simulink model "GAModelTest"  (R2020a)
settings: Solver=FixedStepDiscrete  StartTime=0.0  StopTime=10.0  RelTol=1e-3  EnableMultiTasking=on
model workspace (MAT data in the model file):
  L1 = 0
  L2 = 0
  L3 = 0
  h1 = 0
  l1 = 0
  l2 = 0
  l3 = 0
  l4 = 0
  m1 = 0
  m2 = 0
  m3 = 0
  m4 = 0
values from neighbouring files (symbols this model uses):
  n = 2    [PolynomialFit.m]    (also in extractdata.m = 10)
undefined symbols (not defined in the file or in its folder): lb, ub
settings Model: DataDictionary=ExoskeletonParameters.sldd  Creator=khoi  LastModifiedBy=khoi
settings SolverCC: AutoInsertRateTranBlk=on
settings DataIOCC: SaveOutput=off  SaveTime=off
settings OptimizationCC: DefaultParameterBehavior=Inlined  InlineInvariantSignals=on  EnhancedBackFolding=on  PassReuseOutputArgsAs=Individual arguments  StateBitsets=on  DataBitsets=on  ZeroExternalMemoryAtStartup=off  ZeroInternalMemoryAtStartup=off  NoFixptDivByZeroProtection=on  LifeSpan=1  OptimizeBlockOrder=speed  DifferentSizesBufferReuse=on  EfficientTunableParamExpr=on
settings DebuggingCC: ParameterTunabilityLossMsg=error
settings HardwareCC: ProdBitPerPointer=32  ProdBitPerSizeT=32  ProdBitPerPtrDiffT=32  ProdLargestAtomicFloat=None  ProdIntDivRoundTo=Floor  ProdWordSize=32  ProdHWDeviceType=Generic->Custom
settings SFSimCC: MATLABDynamicMemAlloc=off
settings RTWCC: SystemTargetFile=ert.tlc  TLCOptions=-p0  GenCodeOnly=on  TemplateMakefile=ert_default_tmf  GenerateReport=on  RTWVerbose=off  IncludeHyperlinkInReport=on  LaunchReport=on
settings CodeAppCC: ForceParamTrailComments=on  IgnoreCustomStorageClasses=off  OperatorAnnotations=on  SimulinkDataObjDesc=on  SFDataObjDesc=on  CustomSymbolStrGlobalVar=rt$N$M  CustomSymbolStrType=$N$M  CustomSymbolStrFcn=$N$M$F  CustomSymbolStrMacro=$N$M  InsertBlockDesc=on
settings ERTTargetCC: TargetLangStandard=C99 (ISO)  CodeReplacementLibrary=ISO_C  GenerateSampleERTMain=on  IncludeMdlTerminateFcn=off  SuppressErrorStatus=on  SupportAbsoluteTime=off  PurelyIntegerCode=on  SupportNonFinite=off  SupportComplex=off  InlinedParameterPlacement=NonHierarchical  RootIOFormat=Structure reference  ERTCustomFileTemplate=example_file_process.tlc

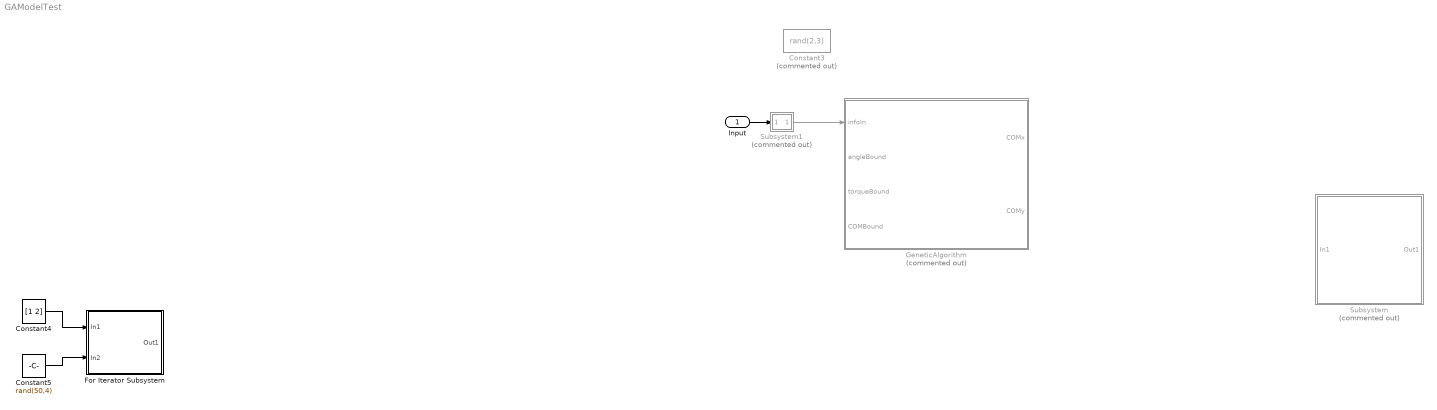
== system GAModelTest ==
  Input : Inport  OutDataTypeStr=Bus: LegSignal
  Constant3 : Constant  Commented=on  Value=rand(2,3)
  Constant4 : Constant  Value=[1 2]
  Constant5 : Constant  Value=rand(50,4)
  For Iterator Subsystem : Subsystem  InitFcn=|  TreatAsAtomicUnit=on  mask{ndec=3, anglb=[1 2 1 1], angub=[5 5 4 3], torlb=[1 1 1 1], torub=[2 2 2 2]}
      | numTotal = (ub-lb)/10^(-ndec) + 1;
      | n = floor(log2(numTotal)) + 1;
      | len = sum(n);
      mask prompts: ndec "Number of decimal place"; anglb "Lower boundary angle"; angub "Upper boundary angle"; torlb "Lower boundary torque"; torub "Upper boundary torque"
  GeneticAlgorithm : Stateflow chart  Commented=on  TreatAsAtomicUnit=on  mask{popSize=50, maxGens=200, probMutation=0.01, crossoverTypeMask=Uniform, probCrossover=0.01, ndec=3, useClamping=on, flagFreq=0, unflagFreq=0, flagPeriod=0, useMaskRepositories=on, maskReposFactor=0, useSUS=on}
      mask prompts: popSize "Population size"; maxGens "Maximum generations"; probMutation "Mutation probability (per bit)"; crossoverTypeMask "Crossover type"; probCrossover "Crossover probability"; ndec "Precision (number of decimal places)"; useClamping "Use clamping"; flagFreq "Flag frequency"; unflagFreq "Unflag frequency"; flagPeriod "Flag period"; useMaskRepositories "Use mask repositories"; maskReposFactor "Factor"; useSUS "Use Stochastic Universal Sampling"
  Subsystem : Subsystem  Commented=on  mask{gainpopup=User-defined, editvalue=2, editvalue_copy=2}
      mask prompts: gainpopup "Gain"; editvalue "Value"; editvalue_copy "Value"
      mask TypeOptions gainpopup: 2 | 5 | User-defined
      mask Callback gainpopup:
      | % Get the mask parameter values. This is a cell
      | %   array of character vectors.
      | maskStr = get_param(gcb,'gainpopup');
      | 
      | % The pop-up menu is the first mask parameter.
      | %   Check the value selected in the pop-up
      | if strcmp(maskStr(1),'U'),
      | 
      |     % Set the visibility of both parameters on when
      |     %   User-defined is selected in the pop-up.
      | 
      |     set_param(gcb,'MaskVisibilities',{'on';'on'}),
      | 
      | else
      | 
      |     % Turn off the visibility of the Value field
      |     %   when User-defined is not selected.
      | 
      |     set_param(gcb,'MaskVisibilities',{'on';'off'}),
      | 
      |     % Set the character vector in the Values field equal to the
      |     % character vector selected in the Gain pop-up menu.
      | 
      |     %maskStr{2}=maskStr{1};
      |     set_param(gcb,'editvalue',maskStr);
      | %     set_param(gcb,'editvalue1',maskStr);
      | end
  Subsystem1 : Subsystem  Commented=on
  wires:
  Input/1 -> Subsystem1/1(In1)
  Subsystem1/1(Out1) -> GeneticAlgorithm/1(infoIn)
  Constant4/1 -> For Iterator Subsystem/1(In1)
  Constant5/1 -> For Iterator Subsystem/2(In2)

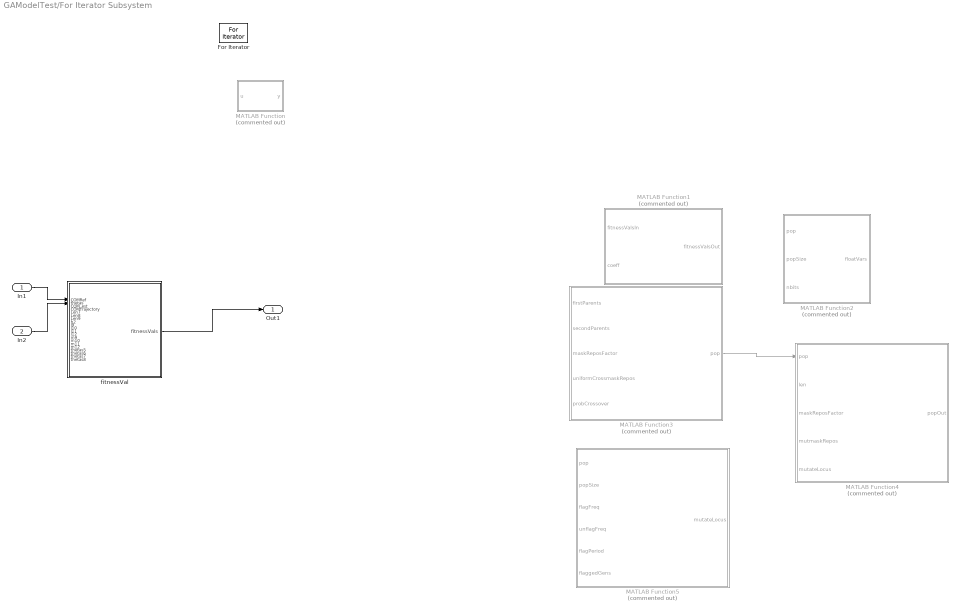
== system GAModelTest/For Iterator Subsystem ==
  In1 : Inport
  In2 : Inport  Port=2
  For Iterator : ForIterator
  MATLAB Function : MATLAB Function  Commented=on  TreatAsAtomicUnit=on
  MATLAB Function1 : MATLAB Function  Commented=on  TreatAsAtomicUnit=on
  MATLAB Function2 : MATLAB Function  Commented=on  TreatAsAtomicUnit=on
  MATLAB Function3 : MATLAB Function  Commented=on  TreatAsAtomicUnit=on
  MATLAB Function4 : MATLAB Function  Commented=on  TreatAsAtomicUnit=on
  MATLAB Function5 : MATLAB Function  Commented=on  TreatAsAtomicUnit=on
  fitnessVal : MATLAB Function  InitFcn=|  TreatAsAtomicUnit=on  mask{Len1=30, h1=10, Len2=400, Len3=500, l1=15, l2=200, l3=250, l4=300, m1=1, m2=5, m3=6, m4=10, useSigmaScaling=on}
      | numTotal = (ub-lb)/10^(-ndec) + 1;
      | n = floor(log2(numTotal)) + 1;
      | len = sum(n);
      mask prompts: Len1 "Feet (mm)"; h1 "Feet offset height (mm)"; Len2 "Lower leg (mm)"; Len3 "Upper leg (mm)"; l1 "Feet (mm)"; l2 "Lower leg (mm)"; l3 "Upper leg (mm)"; l4 "Upper body (mm)"; m1 "Feet (kg)"; m2 "Lower leg (kg)"; m3 "Upper leg (kg)"; m4 "Upper body (kg)"; useSigmaScaling "Use sigma scaling"
  Out1 : Outport
  wires:
  fitnessVal/1(fitnessVals) -> Out1/1
  In1/1 -> fitnessVal/1(COMRef)
  In2/1 -> fitnessVal/2(thetas)
  MATLAB Function3/1(pop) -> MATLAB Function4/1(pop)

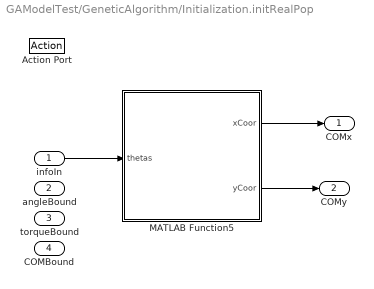
== system GAModelTest/GeneticAlgorithm/Initialization.initRealPop ==
  infoIn : Inport
  angleBound : Inport  Port=2
  torqueBound : Inport  Port=3
  COMBound : Inport  Port=4
  Action Port : ActionPort
      settings: CopyFcn=Stateflow.SLINSF.SimulinkMan.removeBlockPreDeleteFcn  PreDeleteFcn=Stateflow.SLINSF.SimulinkMan.unsafePredeleteFcn
  MATLAB Function5 : MATLAB Function  TreatAsAtomicUnit=on  mask{Len1=30, h1=10, Len2=400, Len3=500, l1=15, l2=200, l3=250, l4=300, m1=1, m2=5, m3=6, m4=10}
      mask prompts: Len1 "Feet (mm)"; h1 "Feet offset height (mm)"; Len2 "Lower leg (mm)"; Len3 "Upper leg (mm)"; l1 "Feet (mm)"; l2 "Lower leg (mm)"; l3 "Upper leg (mm)"; l4 "Upper body (mm)"; m1 "Feet (kg)"; m2 "Lower leg (kg)"; m3 "Upper leg (kg)"; m4 "Upper body (kg)"
  COMx : Outport
  COMy : Outport  Port=2
  wires:
  infoIn/1 -> MATLAB Function5/1(thetas)
  MATLAB Function5/1(xCoor) -> COMx/1
  MATLAB Function5/2(yCoor) -> COMy/1

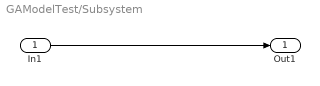
== system GAModelTest/Subsystem ==
  In1 : Inport
  Out1 : Outport
  wires:
  In1/1 -> Out1/1

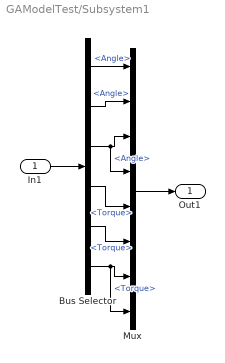
== system GAModelTest/Subsystem1 ==
  In1 : Inport
  Bus Selector : BusSelector  OutputSignals=Hip.Angle,Knee.Angle,Ankle.Angle,Hip.Torque,Knee.Torque,Ankle.Torque
  Mux : Mux  Inputs=8
  Out1 : Outport
  wires:
  Bus Selector/1 -> Mux/1  "<Angle>"
  Bus Selector/2 -> Mux/2  "<Angle>"
  Mux/1 -> Out1/1
  Bus Selector/4 -> Mux/5  "<Torque>"
  Bus Selector/5 -> Mux/6  "<Torque>"
  In1/1 -> Bus Selector/1
  Bus Selector/3 -> Mux/4, Mux/3  "<Angle>"
  Bus Selector/6 -> Mux/7, Mux/8  "<Torque>"

== matlab function GAModelTest/For Iterator Subsystem/MATLAB Function2 ==
  data: pop input; floatVars output; popSize input; nbits input
function floatVars = Decode(pop, popSize, nbits)

cl = [1; cumsum(nbits(1:end-1)+1)];
cu = cumsum(nbits);
floatNum = zeros(popSize, length(nbits));
vars = cell(length(nbits),1);

for i=1:length(nbits)
    vars{i} = pop(:,cl(i):cu(i));
    % gene decoding, with lb = lower bound, ub = upper bound
    % X = X_lb + bin2dec(Xbin)*(X_ub-X_lb)/(2^bitlength-1)
    floatNum(:,i) = lb(i) + bi2de(vars{i},2,'left-msb') ...
        .*(ub(i)-lb(i))./(2.^(nbits(i))-1);
end

floatVars = floatNum;

== matlab function GAModelTest/For Iterator Subsystem/MATLAB Function1 ==
  data: fitnessValsIn input; fitnessValsOut output; coeff input
function fitnessValsOut = SigmaScaling(fitnessValsIn, coeff)

    % Y = output, U = input
    
    sigma=std(fitnessValsIn);
    if sigma~=0
        fitnessValsIn=1+(fitnessValsIn-mean(fitnessValsIn))/...
        (coeff*sigma);
        fitnessValsIn(fitnessValsIn<=0)=0;
    else
        fitnessValsIn=ones(1,popSize);
    end
fitnessValsOut = fitnessValsIn;

== matlab function GAModelTest/For Iterator Subsystem/MATLAB Function3 ==
  data: firstParents input; pop output; secondParents input; maskReposFactor input; uniformCrossmaskRepos input; probCrossover input
function pop = Crossover(firstParents, secondParents, ...
    maskReposFactor, uniformCrossmaskRepos, probCrossover)
    
    % create crossover masks
    temp=floor(rand*len*(maskReposFactor-1));
    masks=uniformCrossmaskRepos(:,temp+1:temp+len);
    
    % determine which parent pairs to leave uncrossed
    reprodIndices=rand(popSize/2,1)<1-probCrossover;
    masks(reprodIndices,:)=false;
    
    % implement crossover
    firstKids=firstParents;
    firstKids(masks)=secondParents(masks);
    secondKids=secondParents;
    secondKids(masks)=firstParents(masks);
    pop=[firstKids; secondKids];

== matlab function GAModelTest/For Iterator Subsystem/MATLAB Function4 ==
  data: pop input; popOut output; len input; maskReposFactor input; mutmaskRepos input; mutateLocus input
function popOut = MaskRepositories(pop, len,...
    maskReposFactor, mutmaskRepos, mutateLocus)
        
    % implement mutation
    temp=floor(rand*len*(maskReposFactor-1));
    masks=mutmaskRepos(:,temp+1:temp+len);

    masks(:,~mutateLocus)=false;
    popOut=xor(pop,masks);

== matlab function GAModelTest/For Iterator Subsystem/MATLAB Function5 ==
  data: pop input; mutateLocus output; popSize input; flagFreq input; unflagFreq input; flagPeriod input; flaggedGens input
function mutateLocus = Clamping(pop, popSize,...
    flagFreq, unflagFreq, flagPeriod, flaggedGens)
    
    bitFreqs=sum(pop)/popSize;

    % perform clamping algorithm
    lociToFlag=abs(0.5-bitFreqs)>(0.5-flagFreq) & flaggedGens<0;
    flaggedGens(lociToFlag)=0;
    lociToUnflag=abs(0.5-bitFreqs)<0.5-unflagFreq ;
    flaggedGens(lociToUnflag)=-1;
    flaggedLoci=flaggedGens>=0;
    flaggedGens(flaggedLoci)=flaggedGens(flaggedLoci)+1;
    mutateLocus=flaggedGens<=flagPeriod;

== stateflow chart GAModelTest/GeneticAlgorithm ==
  state Initialization
    entry:
    crossoverType = crossoverTypeMask - 1;
    % generate chromosome length
    lb = [angleBound(1,:) torqueBound(1,:) COMBound(1)]';
    ub = [angleBound(2,:) torqueBound(2,:) COMBound(2)]';
    numTotal = (ub - lb)/10^(-ndec) + 1;
    nBin = floor(log2(numTotal)) + 1;
    len = sum(nBin);
    pop = InitRealPop(popSize,ub,lb);
    state initRealPop
    state DecisionMaking [commented out]
      (default) -> (junction 192) [commented out] : % 1 => draw uniform crossover and mutation masks from
          | %      a pregenerated repository of randomly generated bits.
          | %      Significantly improves the speed of the code with
          | %      no apparent changes in the behavior of
          | %      the SGA
          | % 0 => generate uniform crossover and mutation
          | %      masks on the fly. Slower.
      (junction 192) -> (junction 199) [commented out] : [useMaskRepositories]
      (junction 192) -> (junction 193) [commented out]
      (junction 199) -> (junction 194) [commented out] : {uniformCrossmaskRepos = rand(popSize/2,(len+1)*maskReposFactor)<0.5;
          | mutmaskRepos = rand(popSize,(len+1)*maskReposFactor)<probMutation;}
      (junction 194) -> (junction 193) [commented out]
      (junction 193) -> (junction 195) [commented out]
    (default) -> initRealPop
  state Fitness
    entry:
    [COMx, COMy] = evalCOMTraj([L1 L2 L3], h1,...
    [l1 l2 l3 l4], [m1 m2 m3 m4], infoIn(1:4));
  state Clamping [commented out]
    during: mutateLocus = performClamping(pop,popSize,flagFreq,unflagFreq,flagPeriod);
  state Clamping1 [commented out]
  state Crossover [commented out]
    entry:
    uniformCrossmaskRepos=rand(popSize/2,(len+1)*maskReposFactor)<0.5;
    (default) -> (junction 98) [commented out] : % create crossover masks
    (junction 98) -> (junction 99) [commented out] : [crossoverType == 0]
    (junction 98) -> (junction 102) [commented out]
    (junction 99) -> (junction 100) [commented out] : {masks = noCrossover(popSize,len);}
    (junction 100) -> (junction 101) [commented out]
    (junction 101) -> (junction 105) [commented out]
    (junction 102) -> (junction 103) [commented out] : [crossoverType == 1]
    (junction 102) -> (junction 106) [commented out] : {2;}
    (junction 103) -> (junction 104) [commented out] : {masks = OnePtCrossover(popSize,len);}
    (junction 104) -> (junction 105) [commented out]
    (junction 105) -> (junction 107) [commented out]
    (junction 107) -> (junction 106) [commented out]
    (junction 106) -> (junction 108) [commented out]
  state Mutation [commented out]
    (default) -> (junction 36) [commented out]
    (junction 36) -> (junction 37) [commented out] : [useMaskRepositories]
    (junction 36) -> (junction 38) [commented out] : {masks=rand(popSize, len)<probMutation;}
    (junction 37) -> (junction 39) [commented out] : {temp=floor(rand*len*(maskReposFactor-1));
        |  masks=mutmaskRepos(:,temp+1:temp+len);}
    (junction 39) -> (junction 38) [commented out]
    (junction 38) -> (junction 40) [commented out]
  state FitnessFunction [commented out]
    entry:
    fitnessVals = fitnessEval(n);
    state EliteFitness [commented out]
  (default) -> Initialization
  Fitness -> Clamping [commented out] : [useClamping]
  Initialization -> Fitness
  Clamping -> (junction 28) [commented out]
  (junction 28) -> Clamping1 [commented out] : [useMaskRepositories]
  data: sf_internal_action_state_placeholder_data local double size=1 =0; fitnessValsIn function_input; y function_output; sigmaCoeff function_input; Ls function_input; h function_input; ls function_input; ms function_input; thetas function_input; xCoor function_output; yCoor function_output; mutateLocus function_output; pop function_input; popSize function_input; flagFreq function_input; unflagFreq function_input; flagPeriod function_input; masks function_output; popSize function_input; len function_input; masks function_output; popSize function_input; len function_input; masks function_output; popSize function_input; len function_input; infoIn input; flaggedGens local double; angleBound input; torqueBound input; COMBound input; lb local size=20; ub local size=20; ndec constant double =3; numTotal local size=20; useClamping parameter double; flagFreq parameter double; unflagFreq parameter double; flagPeriod parameter double; maxGens parameter; maxFitnessHist local; nBin local size=20; popSize parameter; mutateLocus local; maskReposFactor parameter; probMutation parameter; useMaskRepositories parameter; masks local; mutmaskRepos local; uniformCrossmaskRepos local; crossoverType local; crossoverTypeMask parameter; pop local size=[1000 500]; m4 parameter; m3 parameter; m1 parameter; m2 parameter; h1 parameter; COMx output; COMy output; L1 parameter; L2 parameter; L3 parameter; l3 parameter; l1 parameter; l2 parameter; l4 parameter; len local; InitRealPop local
  function y = sigmaScaling(fitnessValsIn,sigmaCoeff):
    | function y = sigmaScaling(fitnessValsIn,sigmaCoeff)
    | sigma=std(fitnessValsIn);
    | if sigma~=0
    |     fitnessValsIn=1+(fitnessValsIn-mean(fitnessValsIn))/...
    |     (sigmaScalingCoeff*sigma);
    |     fitnessValsIn(fitnessValsIn<=0)=0;
    | else
    |     fitnessValsIn=ones(1,popSize);
    | end
    | y = fitnessValsIn;
  function [xCoor, yCoor] = evalCOMTraj(Ls,h,ls,ms,thetas):
    | function [xCoor, yCoor] = evalCOMTraj(Ls,h,ls,ms,thetas)
    | COM_est = COMTrajectory(Ls(1),Ls(2),Ls(3),...
    |                            h,ls(1),ls(2),ls(3),ls(4),...
    |                              ms(1),ms(2),ms(3),ms(4),...
    |                              thetas(1),thetas(2),thetas(3),thetas(4));
    | xCoor = COM_est(1);
    | yCoor = COM_est(2);
  function mutateLocus = performClamping(pop,popSize,flagFreq,unflagFreq,flagPeriod):
    | function mutateLocus = performClamping(pop,popSize,flagFreq,unflagFreq,flagPeriod)
    | 
    | bitFreqs=sum(pop)/popSize;
    | lociToFlag=abs(0.5-bitFreqs)>(0.5-flagFreq) & flaggedGens<0;
    | flaggedGens(lociToFlag)=0;
    | lociToUnflag=abs(0.5-bitFreqs)<0.5-unflagFreq ;
    | flaggedGens(lociToUnflag)=-1;
    | flaggedLoci=flaggedGens>=0;
    | flaggedGens(flaggedLoci)=flaggedGens(flaggedLoci)+1;
    | mutateLocus=flaggedGens<=flagPeriod;
  function masks = uniformCrossover(popSize,len):
    | function masks = uniformCrossover(popSize,len)
    | % mutationOnlycrossmasks
    | masks=false(popSize,len);
  function masks = noCrossover(popSize,len):
    | function masks = noCrossover(popSize,len)
    | % mutationOnlycrossmasks
    | masks=false(popSize,len);
  function masks = OnePtCrossover(popSize,len):
    | function masks = OnePtCrossover(popSize,len)
    | % 1 point crossover
    | masksMat=false(popSize/2, len);
    | temp=ceil(rand(popSize/2,1)*(len-1));
    | for i=1:popSize/2
    |     masksMat(i,1:temp(i))=true;
    | end
    | masks = masksMat;

== matlab function GAModelTest/GeneticAlgorithm/Initialization.initRealPop/MATLAB Function5 ==
  data: h1 parameter; l1 parameter; l2 parameter; l3 parameter; l4 parameter; m1 parameter; m2 parameter; m3 parameter; m4 parameter; thetas input; xCoor output; yCoor output; Len1 parameter; Len2 parameter; Len3 parameter
function [xCoor,yCoor] = evalCOMTraj(h1,...
                           l1,l2,l3,l4,...
                           m1,m2,m3,m4,thetas, Len1, Len2, Len3)
    COM_est = COMTrajectory(Len1,Len2,Len3,h1,...
                           l1,l2,l3,l4,...
                           m1,m2,m3,m4,...
                           thetas(1),thetas(2),thetas(3),thetas(4));
    xCoor = COM_est(1);
    yCoor = COM_est(2);
end

== matlab function GAModelTest/For Iterator Subsystem/MATLAB Function ==
  data: u input; y output
function y = initialization(u)

y = u;

== matlab function GAModelTest/For Iterator Subsystem/fitnessVal ==
  data: COMRef input; h1 parameter; l1 parameter; l2 parameter; l3 parameter; l4 parameter; m1 parameter; m2 parameter; m3 parameter; m4 parameter; Len1 parameter; Len2 parameter; Len3 parameter; thetas input; fitnessVals output; n parameter; ub parameter; lb parameter; useSigmaScaling parameter; COM_est input; COMTrajectory input; Len7 input; Len8 input; Len9 input; h2 input; l9 input; l10 input; l11 input; l12 input; m9 input; m10 input; m11 input; m12 input; thetas5 input; thetas6 input; thetas7 input; thetas8 input
function fitnessVals = fitnessEval(COMRef, h1,...
                           l1,l2,l3,l4,...
                           m1,m2,m3,m4,...
                           Len1,Len2,Len3,...
                           thetas, n, ub, lb, useSigmaScaling,...
    COM_est,  COMTrajectory,Len7,Len8,Len9,h2,...
                           l9,l10,l11,l12,...
                           m9,m10,m11,m12,...
                           thetas5,     thetas6,     thetas7,     thetas8)
    COMRefMat = repmat(COMRef',size(COM_est,1),1);
    fitnessVals = 1./(2*sqrt(dot(COM_est-COMRefMat,COM_est-COMRefMat,2)) + 1);
    if 
    
    else
        
    end
    % encode the real values
    binNum = zeros(popSize,len);
    for i=1:length(n)
        %     gene encoding, with lb = lower bound, ub = upper bound
        %     X_bin = dec2bin( (X-X_lb)*(2^bitlength-1)/(X_ub-X_lb) )
        binNum(:,cl(i):cu(i)) = de2bi(round((fitnessVals(:,i)-lb(i))*(2^(n(i))-1)/(ub(i)-lb(i))),'left-msb');
    end
    
    
    % Conditionally perform sigma scaling.
    % Sigma Scaling is described on pg 168 of M. Mitchell's
    % GA book. It often improves GA performance.
    if useSigmaScaling
        sigma=std(binNum);
        if sigma~=0
            binNum=1+(binNum-mean(binNum))/...
            (sigmaScalingCoeff*sigma);
            binNum(binNum<=0)=0;
        else
            binNum=ones(1,popSize);
        end
    end
    fitnessVals = binNum;
end
